simulink model "steppermotor"  (R2017b)
settings: Solver=ode23tb  StartTime=0.0  StopTime=0.5  FixedStep=Ts  MaxStep=2e-6  EnableMultiTasking=on
PreLoadFcn:
  | assignin('base','Ts',1e-6);
InitFcn:
  | Ts=1e-7;
libraries: powerlib x9, powerlib_meascontrol x2, simulink x1
Description:
  | Copyright 2008-2017 The MathWorks, Inc.
settings Model: ExtModeAutoUpdateStatusClock=off  Creator=MathWorks  LastModifiedBy=Administrator
settings DataIOCC: LimitDataPoints=on  SaveFormat=Array
settings OptimizationCC: ExpressionDepthLimit=2147483647  InitFltsAndDblsToZero=on  LifeSpan=inf
settings DebuggingCC: UnderspecifiedInitializationDetection=Classic  MergeDetectMultiDrivingBlocksExec=none  SignalResolutionControl=TryResolveAllWithWarning  SolverPrmCheckMsg=warning  FcnCallInpInsideContextMsg=warning  StateNameClashWarn=warning  SFUnexpectedBacktrackingDiag=warning  SFNoUnconditionalDefaultTransitionDiag=warning  SFExecutionAtInitializationDiag=none
settings HardwareCC: ProdBitPerPointer=32  ProdBitPerSizeT=32  ProdBitPerPtrDiffT=32  ProdLargestAtomicFloat=None  ProdIntDivRoundTo=Undefined  ProdEndianess=Unspecified  ProdWordSize=32  ProdHWDeviceType=32-bit Generic
settings ModelReferenceCC: PropagateSignalLabelsOutOfModel=off
settings CodeAppCC: StateflowObjectComments=on
settings GRTTargetCC: TargetLangStandard=C89/C90 (ANSI)  GeneratePreprocessorConditionals=Disable all  CombineOutputUpdateFcns=off  GRTInterface=on
settings ConfigComp: CovMetricSettings=dw  CovHtmlReporting=on  CovSaveCumulativeToWorkspaceVar=on  CovSaveSingleToWorkspaceVar=on  CovExternalEMLEnable=off  CovSFcnEnable=off
settings SimscapeCC: SimscapeNormalizeSystem=off

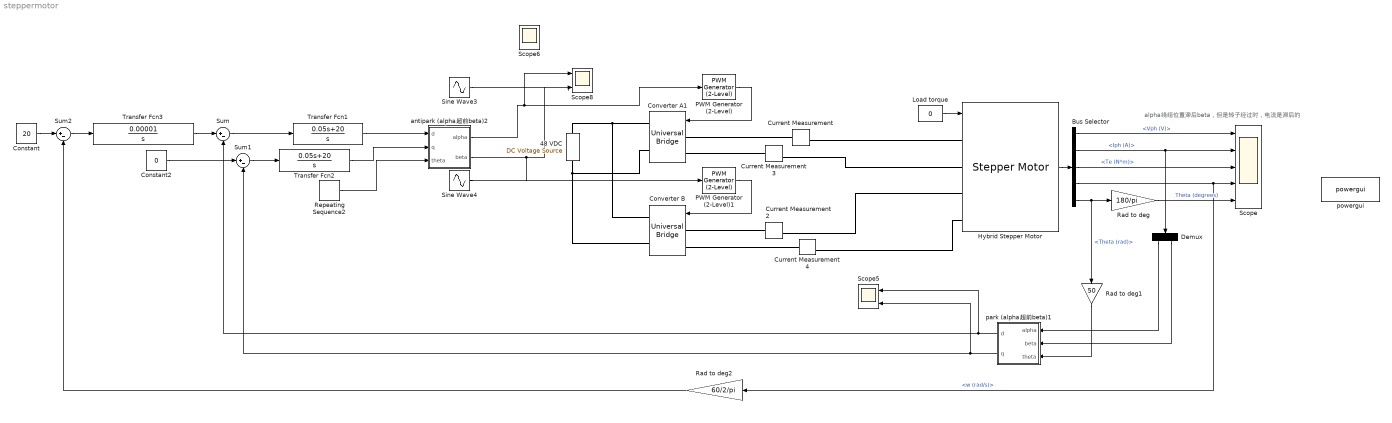
== system steppermotor ==
  note: alpha绕组位置滞后beta，但是转子经过时，电流是滞后的
  48 VDC : powerlib/Electrical Sources/DC Voltage Source  Amplitude=48  Measurements=None
  Bus Selector : BusSelector  OutputSignals=Vph (V),Iph (A),Te (N*m),w (rad/s),Theta (rad)
  Constant : Constant  Value=20
  Constant2 : Constant  Value=0
  Converter A1 : powerlib/Power Electronics/Universal Bridge  Arms=2  SnubberResistance=10000  SnubberCapacitance=inf  Device=MOSFET / Diodes  Ron=1e-3*10  Lon=0  ForwardVoltages="[  0  0  ]"  ForwardVoltage=0  GTOparameters=[ 10e-6 , 20e-6 ]  IGBTparameters=[ 0.5e-6 , 0.5e-6 ]  Measurements=None  Measurements_2=None  converterType=Rectifier
  Converter B : powerlib/Power Electronics/Universal Bridge  Arms=2  SnubberResistance=10000  SnubberCapacitance=inf  Device=MOSFET / Diodes  Ron=1e-3*10  Lon=0  ForwardVoltages="[  0  0  ]"  ForwardVoltage=0  GTOparameters=[ 10e-6 , 20e-6 ]  IGBTparameters=[ 0.5e-6 , 0.5e-6 ]  Measurements=None  Measurements_2=None  converterType=Rectifier
  Current Measurement{,2..4} (4 alike) : powerlib/Measurements/Current Measurement  PhasorSimulation=off  OutputType=Complex  PSBequivalent=0
  Demux : Demux  Outputs=2
  Hybrid Stepper Motor : powerlib/Machines/Stepper Motor  MotorType=Permanent-magnet / Hybrid  NumberOfPhases_1=2  NumberOfPhases_2=3  PresetModel_1=<empty>  PresetModel_2=<empty>  L=1.4e-3  Lmax=10e-3  Lmin=2e-3  R=0.7  Step_angle=1.8  Psim=0.005  Tdm=0.002  J=1.2e-7  B=1e-7*1000  w0=0  pos0=0  TsPowergui=0  TsBlock=-1
      settings: SourceProductName=Simscape Power Systems  SourceProductBaseCode=PS
  Load torque : Constant  Value=0
  PWM Generator (2-Level) : powerlib_meascontrol/Pulse & Signal Generators/PWM Generator (2-Level)  ModulatorType=Single-phase full-bridge (4 pulses)  ModulatorMode=Unsynchronized  Fc=10000  Pc=90  nF=27  MinMax="[ -1  1 ]"  SamplingTechnique=Natural  ModulatingSignals=off  m=0.8  Freq=60  Phase=0  Ts=0  ShowCarrierOutport=off
      settings: SourceProductName=Simscape Power Systems
  PWM Generator (2-Level)1 : powerlib_meascontrol/Pulse & Signal Generators/PWM Generator (2-Level)  ModulatorType=Single-phase full-bridge (4 pulses)  ModulatorMode=Unsynchronized  Fc=10000  Pc=90  nF=27  MinMax="[ -1  1 ]"  SamplingTechnique=Natural  ModulatingSignals=off  m=0.8  Freq=60  Phase=0  Ts=0  ShowCarrierOutport=off
      settings: SourceProductName=Simscape Power Systems
  Rad to deg : Gain  Gain=180/pi
  Rad to deg1 : Gain  Gain=50
  Rad to deg2 : Gain  Gain=60/2/pi
  Repeating Sequence2 : simulink/Sources/Repeating Sequence  rep_seq_t=[0 0.01]  rep_seq_y=[0 2*pi]
  Scope : Scope  NumInputPorts=5
  Scope5 : Scope  NumInputPorts=2
  Scope6 : Scope  NumInputPorts=2
  Scope8 : Scope  NumInputPorts=2
  Sine Wave3 : Sin  Frequency=50*2*pi  SampleTime=0
  Sine Wave4 : Sin  Frequency=50*2*pi  Phase=-pi/2  SampleTime=0
  Sum : Sum  Inputs=|+-
  Sum1 : Sum  Inputs=|+-
  Sum2 : Sum  Inputs=|+-
  Transfer Fcn1 : TransferFcn  Numerator=[0.05 20]  Denominator=[1 0]
  Transfer Fcn2 : TransferFcn  Numerator=[0.05 20]  Denominator=[1 0]
  Transfer Fcn3 : TransferFcn  Numerator=[0.00001]  Denominator=[1 0]
  antipark (alpha超前beta)2 : Subsystem
  park (alpha超前beta)1 : Subsystem
  powergui : powerlib/powergui  SimulationMode=Discrete  SampleTime=Ts  frequency=60  Iterations=50  frequencyindice=0  Pbase=100e6  ErrMax=1e-4  UnitsV=kV  UnitsW=MW  buscounter=0  FunctionMessages=off  echomessages=off  EnableUseOfTLC=off  CurrentSourceSwitches=off  DisableSnubberDevices=off  DisableRonSwitches=off  DisableVfSwitches=off  DisplayEquations=off  SolverType=Tustin/Backward Euler (TBE)  Interpol=off  ExternalGateDelay=off  methode=off  Ts=100  x0status=blocks  SPID=off  SwTol=0  HookPort=off  RestoreLinks=warning  ResistiveCurrentMeasurement=off  Frange=[0:2:500]  Ylog=off  Xlog=on  ShowGrid=off  save=off  variable=ZData  structure=0  ZoomFFT=on  StartTime=0.0  cycles=1  DisplayStyle=1  fundamental=60  FreqAxis=off  MaxFrequency=1000  frequencyindicesteady=1  RmsSteady=1  display=off
  wires:
  Load torque/1 -> Hybrid Stepper Motor/1
  Hybrid Stepper Motor/1 -> Bus Selector/1
  Bus Selector/1 -> Scope/1  "<Vph (V)>"
  Bus Selector/2 -> Scope/2, Demux/1  "<Iph (A)>"
  Bus Selector/3 -> Scope/3  "<Te (N*m)>"
  Bus Selector/4 -> Rad to deg2/1, Scope/4  "<w (rad/s)>"
  Rad to deg/1 -> Scope/5  "Theta (degrees)"
  Bus Selector/5 -> Rad to deg/1, Rad to deg1/1  "<Theta (rad)>"
  PWM Generator (2-Level)1/1 -> Converter B/1
  PWM Generator (2-Level)/1 -> Converter A1/1
  Sine Wave3/1 -> ?
  Sine Wave4/1 -> ?
  Demux/1 -> park (alpha超前beta)1/1(alpha)
  park (alpha超前beta)1/1(d) -> Sum/2, Scope5/1
  park (alpha超前beta)1/2(q) -> Scope5/2, Sum1/2
  Demux/2 -> park (alpha超前beta)1/2(beta)
  Rad to deg1/1 -> park (alpha超前beta)1/3(theta)
  antipark (alpha超前beta)2/1(alpha) -> Scope8/1, PWM Generator (2-Level)/1
  antipark (alpha超前beta)2/2(beta) -> Scope8/2, PWM Generator (2-Level)1/1
  Repeating Sequence2/1 -> antipark (alpha超前beta)2/3(theta)
  Sum/1 -> Transfer Fcn1/1
  Sum1/1 -> Transfer Fcn2/1
  Constant/1 -> Sum2/1
  Constant2/1 -> Sum1/1
  Transfer Fcn1/1 -> antipark (alpha超前beta)2/1(d)
  Transfer Fcn2/1 -> antipark (alpha超前beta)2/2(q)
  Rad to deg2/1 -> Sum2/2
  Sum2/1 -> Transfer Fcn3/1
  Transfer Fcn3/1 -> Sum/1
  connections:
  Current Measurement3/RConn1 -- Hybrid Stepper Motor/LConn2
  Current Measurement2/RConn1 -- Hybrid Stepper Motor/LConn3
  Current Measurement/RConn1 -- Hybrid Stepper Motor/LConn1
  Current Measurement4/RConn1 -- Hybrid Stepper Motor/LConn4
  Converter A1/RConn2 -- Converter B/RConn2 -- 48 VDC/LConn1
  Converter A1/RConn1 -- 48 VDC/RConn1 -- Converter B/RConn1
  Current Measurement3/LConn1 -- Converter A1/LConn2
  Converter B/LConn1 -- Current Measurement2/LConn1
  Current Measurement4/LConn1 -- Converter B/LConn2
  Converter A1/LConn1 -- Current Measurement/LConn1

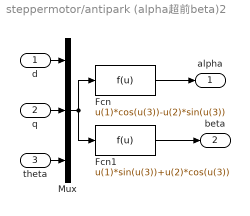
== system steppermotor/antipark (alpha超前beta)2 ==
  d : Inport
  q : Inport  Port=2
  theta : Inport  Port=3
  Fcn : Fcn  Expr=u(1)*cos(u(3))-u(2)*sin(u(3))
  Fcn1 : Fcn  Expr=u(1)*sin(u(3))+u(2)*cos(u(3))
  Mux : Mux  Inputs=3
  alpha : Outport
  beta : Outport  Port=2
  wires:
  Fcn1/1 -> beta/1
  Fcn/1 -> alpha/1
  q/1 -> Mux/2
  d/1 -> Mux/1
  Mux/1 -> Fcn1/1, Fcn/1
  theta/1 -> Mux/3

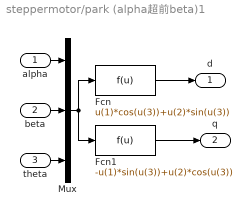
== system steppermotor/park (alpha超前beta)1 ==
  alpha : Inport
  beta : Inport  Port=2
  theta : Inport  Port=3
  Fcn : Fcn  Expr=u(1)*cos(u(3))+u(2)*sin(u(3))
  Fcn1 : Fcn  Expr=-u(1)*sin(u(3))+u(2)*cos(u(3))
  Mux : Mux  Inputs=3
  d : Outport
  q : Outport  Port=2
  wires:
  Fcn1/1 -> q/1
  Fcn/1 -> d/1
  beta/1 -> Mux/2
  alpha/1 -> Mux/1
  Mux/1 -> Fcn1/1, Fcn/1
  theta/1 -> Mux/3
